simulink model "PID_integral"  (R2014a)
settings: Solver=ode45  StartTime=0.0  StopTime=10.0  RelTol=1e-3
settings Model: Creator=York  LastModifiedBy=York

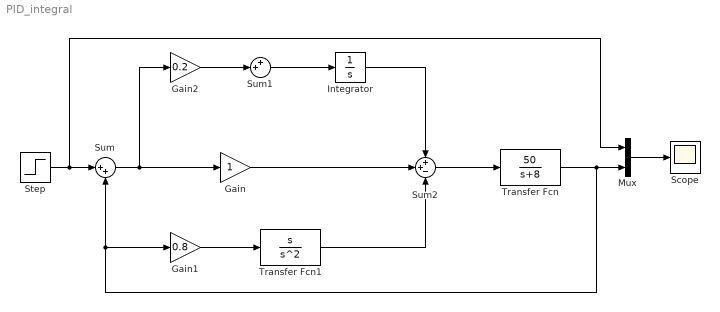
== system PID_integral ==
  Gain : Gain
  Gain1 : Gain  Gain=0.8
  Gain2 : Gain  Gain=0.2
  Integrator : Integrator
  Mux : Mux  Inputs=2
  Scope : Scope
  Step : Step  Time=10  SampleTime=0
  Sum : Sum  Inputs=|++
  Sum1 : Sum  Inputs=++|
  Sum2 : Sum  Inputs=++-
  Transfer Fcn : TransferFcn  Numerator=[50]  Denominator=[1 8]
  Transfer Fcn1 : TransferFcn  Numerator=[1 0]  Denominator=[1 0 0]
  wires:
  Step/1 -> Mux/1, Sum/1
  Gain1/1 -> Transfer Fcn1/1
  Gain/1 -> Sum2/2
  Integrator/1 -> Sum2/1
  Sum1/1 -> Integrator/1
  Gain2/1 -> Sum1/2
  Sum/1 -> Gain2/1, Gain/1
  Sum2/1 -> Transfer Fcn/1
  Transfer Fcn/1 -> Sum/2, Gain1/1, Mux/2
  Mux/1 -> Scope/1
  Transfer Fcn1/1 -> Sum2/3
